simulink model "HVModAL_Fahrzeugmodell"  (R2015b)
settings: Solver=ode1  StartTime=0  StopTime=drp.driving_cycle.tstop  FixedStep=sim_params.Ts  RelTol=1e-5
PreLoadFcn:
  | % Add paths
  | addpath data
  | addpath(genpath('library'))
StartFcn:
  | Simulation.StartTime = tic;
StopFcn:
  | Simulation.DurationTime = toc(Simulation.StartTime);
undefined symbols (not defined in the file or in its folder): Batteries, BMS, BMS_Bat_, C_Nenn_DCDC1, C_Nenn_DCDC2, d2d, DC, DCDC_Converter_efficiency, DcDc_Converters, Dcl, drp, drv, elm, gen, gin, Hdc, hdc, HV, hvb, Hvb, ice, ldc, lib_dcl, lib_hdc, lib_hvb, lib_veh, Link, lossestable, mask_LUT_OCV, mask_LUT_OCV_SOC, mask_LUT_OCV_Temperature, mask_LUT_R, mask_LUT_Rs, mask_LUT_Rs_SOC, mask_LUT_Rs_Temperature, sim_params, speedvec, torquevec, tri, veh, Veh, Vehicle_Chassis
libraries: simulink x29, lib_tri_modules x7, lib_hdc_module x5, lib_gearbox x4, lib_hvb_battery_pack x3, cstblocks x3, PowerLimitBlock x2, MultiCellLibrary x2, lib_aux x1, lib_drv x1, lib_gen x1, lib_elm x1
(part 3 of 7)

== system HVModAL_Fahrzeugmodell/Visualization (Vis)/Subsystem1 ==
  Aux Scope : Scope  NumInputPorts=2
  Auxillaries (aux) : Subsystem
  DC-Link (Dcl) : Subsystem
  DC/DC Converter (hdc) : Subsystem
  DC/DC Scope1 : Scope  NumInputPorts=3
  DC/DC Scope2 : Scope  NumInputPorts=4
  Dcl Scope : Scope  NumInputPorts=4
  Degradation1 : Scope  Commented=on  NumInputPorts=8
  Degradation2 : Scope  Commented=on  NumInputPorts=8
  Demux{1..2,4..5} (4 alike) : Demux  Commented=on  Outputs=3
  Demux3 : Demux  Commented=on  Outputs=8
  Driver (Drv) : Subsystem
  Driver Scope : Scope  NumInputPorts=4
  EMS : Subsystem
  Elm : Subsystem
  Elm Scope : Scope  NumInputPorts=3
  Elm Scope1 : Scope  NumInputPorts=3
  Energy-Disppation Bat1+Bat2 : Scope  NumInputPorts=4
  HV-Batteries (hvb) : Subsystem
  HV-Batteries Scope : Scope  NumInputPorts=6
  Hvb Scope : Scope
  Hvb Scope1 : Scope
  LV-DCDC (ldc) : Subsystem
  Ldc Scope 1 : Scope  NumInputPorts=3
  Ldc Scope 2 : Scope  NumInputPorts=3
  Subsystem1 : Subsystem  Commented=on
  Sum of Elements : Sum  Commented=on  Inputs=+
  Sum of Elements1 : Sum  Commented=on  Inputs=+
  Sum of Elements2 : Sum  Commented=on  Inputs=+
  Terminator{,1..7} (8 alike) : Terminator  Commented=on
  Traction Inverters(Tri) : Subsystem
  Traction Inverters(Tri)- Scope : Scope  NumInputPorts=5
  Veh Scope : Scope  NumInputPorts=5
  Veh Scope 2 : Scope  NumInputPorts=4
  Vehicle (veh) : Subsystem
  wires:
  Vehicle (veh)/4(Veh_F_roll) -> Veh Scope/4  "Veh_F_roll"
  LV-DCDC (ldc)/2(Ldc_P_HvBat_vec) -> Ldc Scope 2/2  "Ldc_P_HvBat_vec"
  Elm/1(Elm_T_el_vec) -> Elm Scope/1  "Elm_T_el"
  Elm/3(Elm_P_losses_vec) -> Elm Scope/3  "Elm_P_losses"
  HV-Batteries (hvb)/12(Hvb_Bat1_Plosses) -> Hvb Scope/1
  DC/DC Converter (hdc)/3(Hdc_P_losses_vec) -> DC/DC Scope2/3  "Hdc_P_losses"
  DC/DC Converter (hdc)/5(Hdc_error_vec) -> DC/DC Scope1/1  "Hdc_error"
  DC/DC Converter (hdc)/6(Hdc_Pmax_vec) -> DC/DC Scope1/2  "Hdc_Pmax"
  Elm/2(Elm_P_actual_vec) -> Elm Scope/2  "Elm_P_actual"
  Traction Inverters(Tri)/5(Tri_atJunction) -> Traction Inverters(Tri)- Scope/5  "Tri_atEndwinding"
  Traction Inverters(Tri)/2(Tri_P_losses) -> Traction Inverters(Tri)- Scope/2  "Tri_P_losses"
  DC/DC Converter (hdc)/4(Hdc_fac_eta_vec) -> DC/DC Scope2/4  "Hdc_fac_eta"
  DC/DC Converter (hdc)/2(Hdc_P_dclink_vec) -> DC/DC Scope2/2  "Hdc_P_dclink"
  HV-Batteries (hvb)/7(Hvb_Bat2_P) -> HV-Batteries Scope/5  "Hvb_Bat2_P"
  HV-Batteries (hvb)/8(Hvb_Bat2_SOC) -> HV-Batteries Scope/6  "Hvb_Bat2_SOC"
  Vehicle (veh)/2(Veh_F_climb) -> Veh Scope/2  "Veh_F_climb"
  Auxillaries (aux)/1(Aux_P_lv_bat) -> Aux Scope/1  "Aux_P_lv_bat"
  HV-Batteries (hvb)/5(Hvb_Bat2_U) -> HV-Batteries Scope/4  "Hvb_Bat2_U"
  HV-Batteries (hvb)/3(Hvb_Bat1_P) -> HV-Batteries Scope/2  "Hvb_Bat1_P"
  HV-Batteries (hvb)/4(Hvb_Bat1_SOC) -> HV-Batteries Scope/3  "Hvb_Bat1_SOC"
  Traction Inverters(Tri)/4(Tri_Pmax) -> Traction Inverters(Tri)- Scope/4  "Tri_Pmax"
  DC-Link (Dcl)/3(Dcl_P_totalwoHdcPdc) -> Dcl Scope/3  "Dcl_P_totalwoHdcPdc"
  HV-Batteries (hvb)/1(Hvb_Bat1_U) -> HV-Batteries Scope/1  "Hvb_Bat1_U"
  Auxillaries (aux)/2(Aux_P_dcLink) -> Aux Scope/2  "Aux_P_dcLink"
  Driver (Drv)/1(fac_pedAcc) -> Driver Scope/1  "fac_pedAcc"
  Vehicle (veh)/3(Veh_F_drive) -> Veh Scope/3  "Veh_F_drive"
  Traction Inverters(Tri)/3(Tri_eta) -> Traction Inverters(Tri)- Scope/3  "Tri_eta"
  LV-DCDC (ldc)/5(Ldc_Pmax_vec) -> Ldc Scope 1/2  "Ldc_Pmax_vec"
  DC/DC Converter (hdc)/1(Hdc_P_bat_vec) -> DC/DC Scope2/1  "Hdc_P_bat"
  LV-DCDC (ldc)/4(Ldc_atJunction_vec) -> Ldc Scope 1/1  "Ldc_atJunction_vec"
  Vehicle (veh)/1(Veh_F_aero) -> Veh Scope/1  "Veh_F_aero"
  Vehicle (veh)/5(Veh_F_acc) -> Veh Scope 2/1, Veh Scope/5  "Veh_F_acc"
  Vehicle (veh)/7(Veh_v_actual) -> Veh Scope 2/3
  Elm/4(Elm1_I_abc) -> Elm Scope1/1  "Elm1_I_abc"
  Elm/6(Elm_at_endWindingsMagnet_vec) -> Elm Scope1/3  "at_end_windingsMagnet_vec"
  Vehicle (veh)/6(Veh_a_actual) -> Veh Scope 2/2
  Vehicle (veh)/8(Veh_v_actual-v_wheel) -> Veh Scope 2/4
  DC-Link (Dcl)/4(Hdc_P_dcLink) -> Dcl Scope/4  "Hdc_P_dcLink"
  DC-Link (Dcl)/1(Dcl_U) -> Dcl Scope/1  "Dcl_U"
  LV-DCDC (ldc)/3(Ldc_P_dcLink) -> Ldc Scope 2/3  "Ldc_P_dcLink"
  LV-DCDC (ldc)/6(Ldc_error_vec) -> Ldc Scope 1/3  "Ldc_error_vec"
  Traction Inverters(Tri)/1(Tri_P_dcLink) -> Traction Inverters(Tri)- Scope/1  "Tri_P_dcLink"
  LV-DCDC (ldc)/1(Ldc_P_Lv_bat) -> Ldc Scope 2/1  "LdcP_Lv_bat"
  Elm/5(Elm_Pmax_vec) -> Elm Scope1/2  "Elm_Pmax_vec"
  DC/DC Converter (hdc)/7(Hdc_at_Junction_vec) -> DC/DC Scope1/3
  Driver (Drv)/2(Emg_T_el_demand) -> Driver Scope/2  "Emg_T_el_demand"
  Driver (Drv)/3(Emg_T_mech_demand) -> Driver Scope/3  "Emg_T_mech_demand"
  DC-Link (Dcl)/2(Dcl_P_total) -> Dcl Scope/2  "Dcl_P_total"
  Driver (Drv)/4(v_cycle(km/h)) -> Driver Scope/4
  EMS/1(Emg_fac_powerDristri_Bat1) -> Energy-Disppation Bat1+Bat2/1  "Emg_fac_powerDristri_Bat1"
  EMS/2(Emg_fac_powerDristri_Bat2) -> Energy-Disppation Bat1+Bat2/2  "Emg_fac_powerDristri_Bat2"
  EMS/6(Emg_T_elDemand_Inv1) -> Energy-Disppation Bat1+Bat2/3  "Emg_T_elDemand_Inv1"
  EMS/7(Emg_T_elDemand_Inv2) -> Energy-Disppation Bat1+Bat2/4  "Emg_T_elDemand_Inv2"
  Vehicle (veh)/9(Veh_Ploss_gearbox) -> Hvb Scope1/1  "Veh_Ploss_gearbox"
  Demux3/1 -> Terminator5/1  "elm1_mot"
  EMS/8(Emg_Degradation) -> Demux3/1
  Demux3/2 -> Terminator4/1  "elm1_gen"
  Demux1/1 -> Sum of Elements/1
  Demux1/2 -> Sum of Elements1/1
  Demux1/3 -> Sum of Elements2/1
  Demux4/1 -> Degradation1/5
  Demux4/2 -> Degradation1/6
  Demux4/3 -> Degradation1/7
  Subsystem1/1(v_deviation(km/h)) -> Degradation2/4, Degradation2/8, Degradation1/4, Degradation1/8
  Demux3/3 -> Terminator6/1  "elm1_mot"
  Demux3/4 -> Terminator7/1  "elm1_gen"
  Demux2/1 -> Degradation2/1
  Demux2/2 -> Degradation2/2
  Demux2/3 -> Degradation2/3
  Demux5/1 -> Degradation2/5
  Demux5/2 -> Degradation2/6
  Demux5/3 -> Degradation2/7
  Sum of Elements/1 -> Degradation1/1
  Sum of Elements1/1 -> Degradation1/2
  Sum of Elements2/1 -> Degradation1/3
  Demux3/5 -> Terminator/1  "tri1_gen"
  Demux3/6 -> Terminator1/1  "DC-Link_gen"
  Demux3/7 -> Terminator2/1
  Demux3/8 -> Terminator3/1

== system HVModAL_Fahrzeugmodell/Energy Manager (Emg)/Battery Control/Driving_Mode ==
  SB_BMS_1 : Inport
  SB_BMS_2 : Inport  Port=2
  SB_BMS_3 : Inport  Port=3
  Veh_v_actual : Inport  Port=4
  Tri_BusSW : Inport  Port=5
  "Aux_BusSW " : Inport  Port=6
  Enable : EnablePort
  Merge : Merge  Inputs=5
  Range_extender 1 : Subsystem  Commented=on  TreatAsAtomicUnit=on
  Range_extender 2 : Subsystem  TreatAsAtomicUnit=on
  Strategy_Maximiziation_Available_Batterypower : Subsystem  TreatAsAtomicUnit=on
  Strategy_Maximiziation_Driving_Range1 : Subsystem  Commented=on  TreatAsAtomicUnit=on
  Strategy_Minimization_Current_Trip_Costs : Subsystem  TreatAsAtomicUnit=on
  Strategy_Minimization_LifeCycleCosts : Subsystem  TreatAsAtomicUnit=on
  Switch Case : SwitchCase  CaseConditions={2, 3, 4,5}
  n_Power_Distribution_Strategy : Constant  Value=5
  vector_PowerDistribution : Outport
  case : Outport  Port=2
  I_rex : Outport  Port=3
  wires:
  Merge/1 -> vector_PowerDistribution/1
  Switch Case/1 -> Strategy_Minimization_Current_Trip_Costs/Action
  Switch Case/2 -> Strategy_Minimization_LifeCycleCosts/Action
  Switch Case/3 -> Strategy_Maximiziation_Driving_Range1/Action
  Switch Case/5 -> Strategy_Maximiziation_Available_Batterypower/Action
  SB_BMS_3/1 -> Range_extender 2/3(SB_BMS_3), Strategy_Maximiziation_Driving_Range1/3(SB_BMS_3), Strategy_Maximiziation_Available_Batterypower/3(SB_BMS_3)
  SB_BMS_2/1 -> Range_extender 2/2(SB_BMS_2), Strategy_Maximiziation_Driving_Range1/2(SB_BMS_2), Strategy_Maximiziation_Available_Batterypower/2(SB_BMS_2)
  SB_BMS_1/1 -> Range_extender 2/1(SB_BMS_1), Strategy_Maximiziation_Driving_Range1/1(SB_BMS_1), Strategy_Maximiziation_Available_Batterypower/1(SB_BMS_1)
  n_Power_Distribution_Strategy/1 -> case/1, Switch Case/1
  Strategy_Minimization_LifeCycleCosts/1(vector_PowerDistribution) -> Merge/3
  Strategy_Maximiziation_Available_Batterypower/1(vector_PowerDistribution) -> Merge/1
  Strategy_Maximiziation_Driving_Range1/1(vector_PowerDistribution) -> Merge/4
  Strategy_Minimization_Current_Trip_Costs/1(vector_PowerDistribution) -> Merge/2
  ? -> ?
  Switch Case/4 -> Range_extender 2/Action
  Range_extender 2/1(vector_PowerDistribution) -> Merge/5
  Veh_v_actual/1 -> Range_extender 2/4(Veh_v_actual)
  Range_extender 2/2(I_rex) -> I_rex/1
  Tri_BusSW/1 -> Range_extender 2/5(Tri_BusSW)
  "Aux_BusSW "/1 -> Range_extender 2/6("Aux_BusSW ")

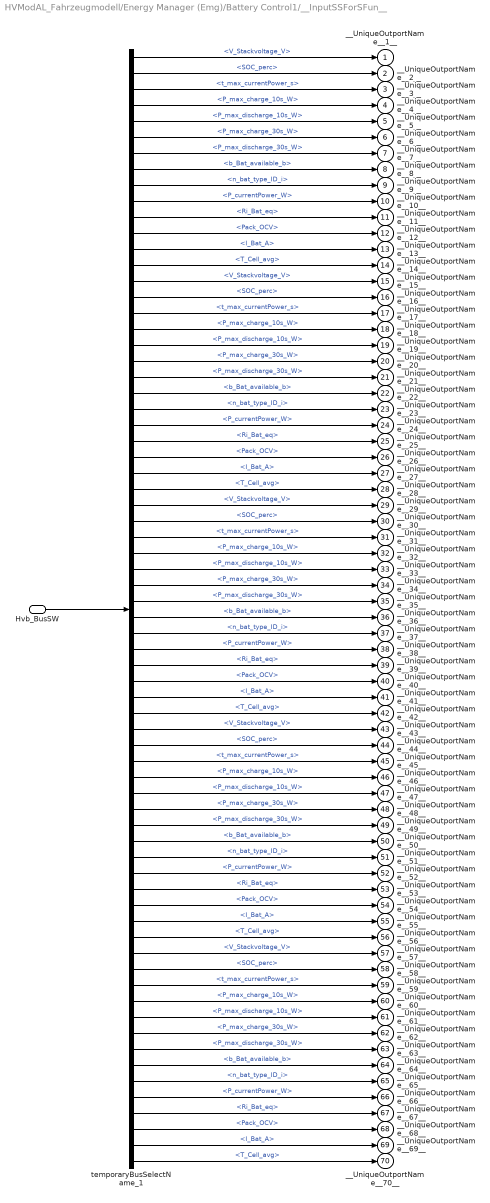
== system HVModAL_Fahrzeugmodell/Energy Manager (Emg)/Battery Control1/__InputSSForSFun__ ==
  Hvb_BusSW : Inport
  temporaryBusSelectName_1 : BusSelector  OutputSignals=SB_Bat1.V_Stackvoltage_V,SB_Bat1.SOC_perc,SB_Bat1.t_max_currentPower_s,SB_Bat1.P_max_charge_10s_W,SB_Bat1.P_max_discharge_10s_W,SB_Bat1.P_max_charge_30s_W,SB_Bat1.P_max_discharge_30s_W,SB_Bat1.b_Bat_available_b,SB_Bat1.n_bat_type_ID_i,SB_Bat1.P_currentPower_W,SB_Bat1.Ri_Bat_eq,SB_Bat1.Pack_OCV,SB_Bat1.I_Bat_A,SB_Bat1.T_Cell_avg,SB_Bat2.V_Stackvoltage_V,SB_Bat2.SOC_perc,SB_Bat2.t_max_currentPower_s,SB_Bat2.P_max_charge_10s_W,SB_Bat2.P_max_discharge_10s_W,SB_Bat2.P_max_charge_30s_W,SB_Bat2.P_max_discharge_30s_W,SB_Bat2.b_Bat_available_b,SB_Bat2.n_bat_type_ID_i,SB_Bat2.P_currentPower_W,SB_Bat2.Ri_Bat_eq,SB_Bat2.Pack_OCV,SB_Bat2.I_Bat_A,SB_Bat2.T_Cell_avg,SB_Bat3.V_Stackvoltage_V,SB_Bat3.SOC_perc,SB_Bat3.t_max_currentPower_s,SB_Bat3.P_max_charge_10s_W,SB_Bat3.P_max_discharge_10s_W,SB_Bat3.P_max_charge_30s_W,SB_Bat3.P_max_discharge_30s_W,SB_Bat3.b_Bat_available_b,SB_Bat3.n_bat_type_ID_i,SB_Bat3.P_currentPower_W,SB_Bat3.Ri_Bat_eq,SB_Bat3.Pack_OCV,SB_Bat3.I_Bat_A,SB_Bat3.T_Cell_avg,SB_Bat4.V_Stackvoltage_V,SB_Bat4.SOC_perc,SB_Bat4.t_max_currentPower_s,SB_Bat4.P_max_charge_10s_W,SB_Bat4.P_max_discharge_10s_W,SB_Bat4.P_max_charge_30s_W,SB_Bat4.P_max_discharge_30s_W,SB_Bat4.b_Bat_available_b,SB_Bat4.n_bat_type_ID_i,SB_Bat4.P_currentPower_W,SB_Bat4.Ri_Bat_eq,SB_Bat4.Pack_OCV,SB_Bat4.I_Bat_A,SB_Bat4.T_Cell_avg,SB_Bat5.V_Stackvoltage_V,SB_Bat5.SOC_perc,SB_Bat5.t_max_currentPower_s,SB_Bat5.P_max_charge_10s_W,SB_Bat5.P_max_discharge_10s_W,SB_Bat5.P_max_charge_30s_W,SB_Bat5.P_max_discharge_30s_W,SB_Bat5.b_Bat_available_b,SB_Bat5.n_bat_type_ID_i,SB_Bat5.P_currentPower_W,SB_Bat5.Ri_Bat_eq,SB_Bat5.Pack_OCV,SB_Bat5.I_Bat_A,SB_Bat5.T_Cell_avg
  __UniqueOutportName__1__ : Outport
  __UniqueOutportName__2__ : Outport  Port=2
  __UniqueOutportName__3__ : Outport  Port=3
  __UniqueOutportName__4__ : Outport  Port=4
  __UniqueOutportName__5__ : Outport  Port=5
  __UniqueOutportName__6__ : Outport  Port=6
  __UniqueOutportName__7__ : Outport  Port=7
  __UniqueOutportName__8__ : Outport  Port=8
  __UniqueOutportName__9__ : Outport  Port=9
  __UniqueOutportName__10__ : Outport  Port=10
  __UniqueOutportName__11__ : Outport  Port=11
  __UniqueOutportName__12__ : Outport  Port=12
  __UniqueOutportName__13__ : Outport  Port=13
  __UniqueOutportName__14__ : Outport  Port=14
  __UniqueOutportName__15__ : Outport  Port=15
  __UniqueOutportName__16__ : Outport  Port=16
  __UniqueOutportName__17__ : Outport  Port=17
  __UniqueOutportName__18__ : Outport  Port=18
  __UniqueOutportName__19__ : Outport  Port=19
  __UniqueOutportName__20__ : Outport  Port=20
  __UniqueOutportName__21__ : Outport  Port=21
  __UniqueOutportName__22__ : Outport  Port=22
  __UniqueOutportName__23__ : Outport  Port=23
  __UniqueOutportName__24__ : Outport  Port=24
  __UniqueOutportName__25__ : Outport  Port=25
  __UniqueOutportName__26__ : Outport  Port=26
  __UniqueOutportName__27__ : Outport  Port=27
  __UniqueOutportName__28__ : Outport  Port=28
  __UniqueOutportName__29__ : Outport  Port=29
  __UniqueOutportName__30__ : Outport  Port=30
  __UniqueOutportName__31__ : Outport  Port=31
  __UniqueOutportName__32__ : Outport  Port=32
  __UniqueOutportName__33__ : Outport  Port=33
  __UniqueOutportName__34__ : Outport  Port=34
  __UniqueOutportName__35__ : Outport  Port=35
  __UniqueOutportName__36__ : Outport  Port=36
  __UniqueOutportName__37__ : Outport  Port=37
  __UniqueOutportName__38__ : Outport  Port=38
  __UniqueOutportName__39__ : Outport  Port=39
  __UniqueOutportName__40__ : Outport  Port=40
  __UniqueOutportName__41__ : Outport  Port=41
  __UniqueOutportName__42__ : Outport  Port=42
  __UniqueOutportName__43__ : Outport  Port=43
  __UniqueOutportName__44__ : Outport  Port=44
  __UniqueOutportName__45__ : Outport  Port=45
  __UniqueOutportName__46__ : Outport  Port=46
  __UniqueOutportName__47__ : Outport  Port=47
  __UniqueOutportName__48__ : Outport  Port=48
  __UniqueOutportName__49__ : Outport  Port=49
  __UniqueOutportName__50__ : Outport  Port=50
  __UniqueOutportName__51__ : Outport  Port=51
  __UniqueOutportName__52__ : Outport  Port=52
  __UniqueOutportName__53__ : Outport  Port=53
  __UniqueOutportName__54__ : Outport  Port=54
  __UniqueOutportName__55__ : Outport  Port=55
  __UniqueOutportName__56__ : Outport  Port=56
  __UniqueOutportName__57__ : Outport  Port=57
  __UniqueOutportName__58__ : Outport  Port=58
  __UniqueOutportName__59__ : Outport  Port=59
  __UniqueOutportName__60__ : Outport  Port=60
  __UniqueOutportName__61__ : Outport  Port=61
  __UniqueOutportName__62__ : Outport  Port=62
  __UniqueOutportName__63__ : Outport  Port=63
  __UniqueOutportName__64__ : Outport  Port=64
  __UniqueOutportName__65__ : Outport  Port=65
  __UniqueOutportName__66__ : Outport  Port=66
  __UniqueOutportName__67__ : Outport  Port=67
  __UniqueOutportName__68__ : Outport  Port=68
  __UniqueOutportName__69__ : Outport  Port=69
  __UniqueOutportName__70__ : Outport  Port=70
  wires:
  Hvb_BusSW/1 -> temporaryBusSelectName_1/1
  temporaryBusSelectName_1/1 -> __UniqueOutportName__1__/1  "<V_Stackvoltage_V>"
  temporaryBusSelectName_1/2 -> __UniqueOutportName__2__/1  "<SOC_perc>"
  temporaryBusSelectName_1/3 -> __UniqueOutportName__3__/1  "<t_max_currentPower_s>"
  temporaryBusSelectName_1/4 -> __UniqueOutportName__4__/1  "<P_max_charge_10s_W>"
  temporaryBusSelectName_1/5 -> __UniqueOutportName__5__/1  "<P_max_discharge_10s_W>"
  temporaryBusSelectName_1/6 -> __UniqueOutportName__6__/1  "<P_max_charge_30s_W>"
  temporaryBusSelectName_1/7 -> __UniqueOutportName__7__/1  "<P_max_discharge_30s_W>"
  temporaryBusSelectName_1/8 -> __UniqueOutportName__8__/1  "<b_Bat_available_b>"
  temporaryBusSelectName_1/9 -> __UniqueOutportName__9__/1  "<n_bat_type_ID_i>"
  temporaryBusSelectName_1/10 -> __UniqueOutportName__10__/1  "<P_currentPower_W>"
  temporaryBusSelectName_1/11 -> __UniqueOutportName__11__/1  "<Ri_Bat_eq>"
  temporaryBusSelectName_1/12 -> __UniqueOutportName__12__/1  "<Pack_OCV>"
  temporaryBusSelectName_1/13 -> __UniqueOutportName__13__/1  "<I_Bat_A>"
  temporaryBusSelectName_1/14 -> __UniqueOutportName__14__/1  "<T_Cell_avg>"
  temporaryBusSelectName_1/15 -> __UniqueOutportName__15__/1  "<V_Stackvoltage_V>"
  temporaryBusSelectName_1/16 -> __UniqueOutportName__16__/1  "<SOC_perc>"
  temporaryBusSelectName_1/17 -> __UniqueOutportName__17__/1  "<t_max_currentPower_s>"
  temporaryBusSelectName_1/18 -> __UniqueOutportName__18__/1  "<P_max_charge_10s_W>"
  temporaryBusSelectName_1/19 -> __UniqueOutportName__19__/1  "<P_max_discharge_10s_W>"
  temporaryBusSelectName_1/20 -> __UniqueOutportName__20__/1  "<P_max_charge_30s_W>"
  temporaryBusSelectName_1/21 -> __UniqueOutportName__21__/1  "<P_max_discharge_30s_W>"
  temporaryBusSelectName_1/22 -> __UniqueOutportName__22__/1  "<b_Bat_available_b>"
  temporaryBusSelectName_1/23 -> __UniqueOutportName__23__/1  "<n_bat_type_ID_i>"
  temporaryBusSelectName_1/24 -> __UniqueOutportName__24__/1  "<P_currentPower_W>"
  temporaryBusSelectName_1/25 -> __UniqueOutportName__25__/1  "<Ri_Bat_eq>"
  temporaryBusSelectName_1/26 -> __UniqueOutportName__26__/1  "<Pack_OCV>"
  temporaryBusSelectName_1/27 -> __UniqueOutportName__27__/1  "<I_Bat_A>"
  temporaryBusSelectName_1/28 -> __UniqueOutportName__28__/1  "<T_Cell_avg>"
  temporaryBusSelectName_1/29 -> __UniqueOutportName__29__/1  "<V_Stackvoltage_V>"
  temporaryBusSelectName_1/30 -> __UniqueOutportName__30__/1  "<SOC_perc>"
  temporaryBusSelectName_1/31 -> __UniqueOutportName__31__/1  "<t_max_currentPower_s>"
  temporaryBusSelectName_1/32 -> __UniqueOutportName__32__/1  "<P_max_charge_10s_W>"
  temporaryBusSelectName_1/33 -> __UniqueOutportName__33__/1  "<P_max_discharge_10s_W>"
  temporaryBusSelectName_1/34 -> __UniqueOutportName__34__/1  "<P_max_charge_30s_W>"
  temporaryBusSelectName_1/35 -> __UniqueOutportName__35__/1  "<P_max_discharge_30s_W>"
  temporaryBusSelectName_1/36 -> __UniqueOutportName__36__/1  "<b_Bat_available_b>"
  temporaryBusSelectName_1/37 -> __UniqueOutportName__37__/1  "<n_bat_type_ID_i>"
  temporaryBusSelectName_1/38 -> __UniqueOutportName__38__/1  "<P_currentPower_W>"
  temporaryBusSelectName_1/39 -> __UniqueOutportName__39__/1  "<Ri_Bat_eq>"
  temporaryBusSelectName_1/40 -> __UniqueOutportName__40__/1  "<Pack_OCV>"
  temporaryBusSelectName_1/41 -> __UniqueOutportName__41__/1  "<I_Bat_A>"
  temporaryBusSelectName_1/42 -> __UniqueOutportName__42__/1  "<T_Cell_avg>"
  temporaryBusSelectName_1/43 -> __UniqueOutportName__43__/1  "<V_Stackvoltage_V>"
  temporaryBusSelectName_1/44 -> __UniqueOutportName__44__/1  "<SOC_perc>"
  temporaryBusSelectName_1/45 -> __UniqueOutportName__45__/1  "<t_max_currentPower_s>"
  temporaryBusSelectName_1/46 -> __UniqueOutportName__46__/1  "<P_max_charge_10s_W>"
  temporaryBusSelectName_1/47 -> __UniqueOutportName__47__/1  "<P_max_discharge_10s_W>"
  temporaryBusSelectName_1/48 -> __UniqueOutportName__48__/1  "<P_max_charge_30s_W>"
  temporaryBusSelectName_1/49 -> __UniqueOutportName__49__/1  "<P_max_discharge_30s_W>"
  temporaryBusSelectName_1/50 -> __UniqueOutportName__50__/1  "<b_Bat_available_b>"
  temporaryBusSelectName_1/51 -> __UniqueOutportName__51__/1  "<n_bat_type_ID_i>"
  temporaryBusSelectName_1/52 -> __UniqueOutportName__52__/1  "<P_currentPower_W>"
  temporaryBusSelectName_1/53 -> __UniqueOutportName__53__/1  "<Ri_Bat_eq>"
  temporaryBusSelectName_1/54 -> __UniqueOutportName__54__/1  "<Pack_OCV>"
  temporaryBusSelectName_1/55 -> __UniqueOutportName__55__/1  "<I_Bat_A>"
  temporaryBusSelectName_1/56 -> __UniqueOutportName__56__/1  "<T_Cell_avg>"
  temporaryBusSelectName_1/57 -> __UniqueOutportName__57__/1  "<V_Stackvoltage_V>"
  temporaryBusSelectName_1/58 -> __UniqueOutportName__58__/1  "<SOC_perc>"
  temporaryBusSelectName_1/59 -> __UniqueOutportName__59__/1  "<t_max_currentPower_s>"
  temporaryBusSelectName_1/60 -> __UniqueOutportName__60__/1  "<P_max_charge_10s_W>"
  temporaryBusSelectName_1/61 -> __UniqueOutportName__61__/1  "<P_max_discharge_10s_W>"
  temporaryBusSelectName_1/62 -> __UniqueOutportName__62__/1  "<P_max_charge_30s_W>"
  temporaryBusSelectName_1/63 -> __UniqueOutportName__63__/1  "<P_max_discharge_30s_W>"
  temporaryBusSelectName_1/64 -> __UniqueOutportName__64__/1  "<b_Bat_available_b>"
  temporaryBusSelectName_1/65 -> __UniqueOutportName__65__/1  "<n_bat_type_ID_i>"
  temporaryBusSelectName_1/66 -> __UniqueOutportName__66__/1  "<P_currentPower_W>"
  temporaryBusSelectName_1/67 -> __UniqueOutportName__67__/1  "<Ri_Bat_eq>"
  temporaryBusSelectName_1/68 -> __UniqueOutportName__68__/1  "<Pack_OCV>"
  temporaryBusSelectName_1/69 -> __UniqueOutportName__69__/1  "<I_Bat_A>"
  temporaryBusSelectName_1/70 -> __UniqueOutportName__70__/1  "<T_Cell_avg>"

== system HVModAL_Fahrzeugmodell/Energy Manager (Emg)/Battery Control1/__OutputSSForSFun__ ==
  __UniqueInportName__1__ : Inport
  Emg_fac_powerDistribution_vec : Outport
  wires:
  __UniqueInportName__1__/1 -> Emg_fac_powerDistribution_vec/1  "Emg_fac_powerDistribution_vec"

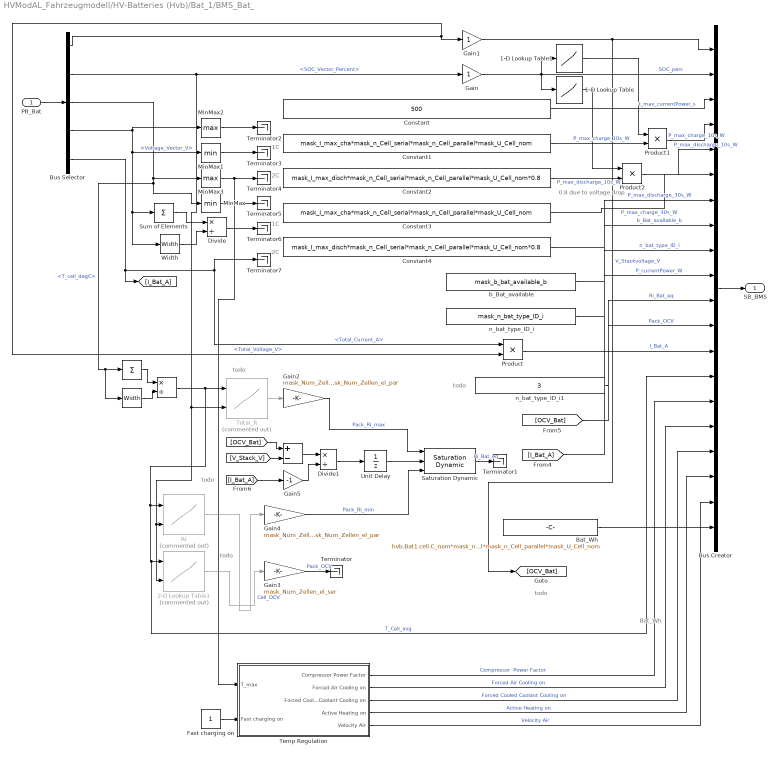
== system HVModAL_Fahrzeugmodell/HV-Batteries (Hvb)/Bat_1/BMS_Bat_ ==
  note: Bat_Wh
  note: 0.8 due to voltage drop
  note: todo
  note: 1C
  note: 2C
  note: 1C
  note: 2C
  note: todo
  note: todo
  note: todo
  note: todo
  PB_Bat : Inport
  " " : Product  Inputs=*/
  " " : Sum  Inputs=+
  " " : Width
  " " : Sum  Inputs=+-
  1-D Lookup Table : Lookup_n-D  NumberOfTableDimensions=1  BreakpointsForDimension1=[0,10,20,40,60,80,100]  Table=[0,0.5,0.8,1,1,1,1]  InternalRulePriority=Speed  RndMeth=Simplest  InputSameDT=on
  1-D Lookup Table1 : Lookup_n-D  NumberOfTableDimensions=1  BreakpointsForDimension1=[0 20 40 60 80 100]  Table=[1 1 1 1 0.7 0]  InternalRulePriority=Speed  RndMeth=Simplest  InputSameDT=on
  2-D Lookup Table1 : Lookup_n-D  Commented=on  BreakpointsForDimension1=mask_LUT_OCV_Temperature  BreakpointsForDimension2=mask_LUT_OCV_SOC  Table=mask_LUT_OCV  InternalRulePriority=Speed  RndMeth=Simplest  InputSameDT=on
  Bat_Wh : Constant  Value=hvb.Bat1.cell.C_nom*mask_n_Cell_serial*mask_n_Cell_parallel*mask_U_Cell_nom
  Bus Creator : BusCreator  Inputs=20
  Bus Selector : BusSelector  OutputSignals=Total_Voltage_V,SOC_Vector_Percent,T_cell_degC,Voltage_Vector_V,Total_Current_A
  Constant : Constant  Value=500
  Constant1 : Constant  Value=mask_I_max_cha*mask_n_Cell_serial*mask_n_Cell_parallel*mask_U_Cell_nom
  Constant2 : Constant  Value=mask_I_max_disch*mask_n_Cell_serial*mask_n_Cell_parallel*mask_U_Cell_nom*0.8
  Constant3 : Constant  Value=mask_I_max_cha*mask_n_Cell_serial*mask_n_Cell_parallel*mask_U_Cell_nom
  Constant4 : Constant  Value=mask_I_max_disch*mask_n_Cell_serial*mask_n_Cell_parallel*mask_U_Cell_nom*0.8
  Divide : Product  Inputs=*/
  Divide1 : Product  Inputs=*/
  Fast charging on : Constant
  Gain : Gain
  Gain1 : Gain
  Gain2 : Gain  Gain=mask_Num_Zellen_el_ser/mask_Num_Zellen_el_par
  Gain3 : Gain  Gain=mask_Num_Zellen_el_ser
  Gain4 : Gain  Gain=mask_Num_Zellen_el_ser/mask_Num_Zellen_el_par
  Gain5 : Gain  Gain=-1
  MinMax : MinMax
  MinMax1 : MinMax
  MinMax2 : MinMax  Function=max
  MinMax3 : MinMax  Function=max
  Product : Product  RndMeth=Zero
  Product1 : Product  RndMeth=Zero
  Product2 : Product  RndMeth=Zero
  Ri : Lookup_n-D  Commented=on  BreakpointsForDimension1=mask_LUT_Rs_Temperature  BreakpointsForDimension2=mask_LUT_Rs_SOC  Table=mask_LUT_Rs  InternalRulePriority=Speed  RndMeth=Simplest  InputSameDT=on
  Saturation Dynamic : simulink/Discontinuities/Saturation Dynamic  OutMin=[]  OutMax=[]  OutDataTypeStr=Inherit: Same as second input  OutDataType=fixdt(1, 16)  OutScaling=2^-10  DoSatur=off
  Sum of Elements : Sum  Inputs=+
  Temp Regulation : Subsystem
  Terminator{,1..7} (8 alike) : Terminator
  Total_R : Lookup_n-D  Commented=on  BreakpointsForDimension1=mask_LUT_Rs_Temperature  BreakpointsForDimension2=mask_LUT_Rs_SOC  Table=mask_LUT_R  InternalRulePriority=Speed  RndMeth=Simplest  InputSameDT=on
  Unit Delay : UnitDelay  InitialCondition=0.1  SampleTime=-1
  Width : Width
  b_Bat_available : Constant  Value=mask_b_bat_available_b
  n_bat_type_ID_i : Constant  Value=mask_n_bat_type_ID_i
  n_bat_type_ID_i1 : Constant  Value=3
  SB_BMS : Outport
  wires:
  Gain1/1 -> [OCV_Bat], Bus Creator/1  "V_Stackvoltage_V"
  n_bat_type_ID_i/1 -> Bus Creator/9  "n_bat_type_ID_i"
  b_Bat_available/1 -> Bus Creator/8  "b_Bat_available_b"
  Constant4/1 -> Bus Creator/7  "P_max_discharge_30s_W"
  Constant3/1 -> Bus Creator/6  "P_max_charge_30s_W"
  Constant2/1 -> Product2/2  "P_max_discharge_10s_W"
  Constant1/1 -> Product1/2  "P_max_charge_10s_W"
  Constant/1 -> Bus Creator/3  "t_max_currentPower_s"
  Bus Selector/5 -> [I_Bat_A], Terminator7/1, Product/1  "<Total_Current_A>"
  Bus Selector/4 -> MinMax2/1, MinMax1/1, Sum of Elements/1, Width/1  "<Voltage_Vector_V>"
  Bus Selector/3 -> " "/1, " "/1, MinMax/1, MinMax3/1  "<T_cell_degC>"
  Bus Selector/1 -> Gain1/1, Product/2  "<Total_Voltage_V>"
  Divide/1 -> Terminator6/1
  Width/1 -> Divide/2
  Sum of Elements/1 -> Divide/1
  MinMax3/1 -> Temp Regulation/1(T_max), Terminator4/1
  MinMax2/1 -> Terminator2/1
  MinMax1/1 -> Terminator3/1
  MinMax/1 -> Terminator5/1
  Gain/1 -> 1-D Lookup Table/1, 1-D Lookup Table1/1, Bus Creator/2  "SOC_perc"
  Bus Creator/1 -> SB_BMS/1
  PB_Bat/1 -> Bus Selector/1
  Product/1 -> Bus Creator/10  "P_currentPower_W"
  Unit Delay/1 -> Saturation Dynamic/2
  [OCV_Bat] -> Bus Creator/12  "Pack_OCV"
  Saturation Dynamic/1 -> Terminator1/1  "Ri_Bat_eq"
  Gain5/1 -> Divide1/2
  " "/1 -> Divide1/1
  [V_Stack_V] -> " "/2
  [OCV_Bat] -> " "/1
  [I_Bat_A] -> Gain5/1
  Divide1/1 -> Unit Delay/1
  [I_Bat_A] -> Bus Creator/13  "I_Bat_A"
  Gain4/1 -> Saturation Dynamic/3  "Pack_Ri_min"
  Ri/1 -> Gain4/1
  Gain3/1 -> Terminator/1  "Pack_OCV"
  Gain2/1 -> Saturation Dynamic/1  "Pack_Ri_max"
  " "/1 -> Ri/1, Bus Creator/14, 2-D Lookup Table1/1, Total_R/1  "T_Cell_avg"
  2-D Lookup Table1/1 -> Gain3/1  "Cell_OCV"
  Total_R/1 -> Gain2/1
  Bus Selector/2 -> Ri/2, 2-D Lookup Table1/2, Total_R/2, Gain/1  "<SOC_Vector_Percent>"
  " "/1 -> " "/2
  " "/1 -> " "/1
  n_bat_type_ID_i1/1 -> Bus Creator/11  "Ri_Bat_eq"
  Product1/1 -> Bus Creator/4  "P_max_charge_10s_W"
  Product2/1 -> Bus Creator/5  "P_max_discharge_10s_W"
  1-D Lookup Table1/1 -> Product1/1
  1-D Lookup Table/1 -> Product2/1
  Temp Regulation/2(Forced Air Cooling on) -> Bus Creator/16  "Forced Air Cooling on"
  Temp Regulation/3(Forced Cooled Coolant Cooling on) -> Bus Creator/17  "Forced Cooled Coolant Cooling on"
  Fast charging on/1 -> Temp Regulation/2(Fast charging on)
  Temp Regulation/4(Active Heating on) -> Bus Creator/18  "Active Heating on"
  Temp Regulation/1(Compressor Power Factor) -> Bus Creator/15  "Compressor  Power Factor"
  Temp Regulation/5(Velocity Air) -> Bus Creator/19  "Velocity Air"
  Bat_Wh/1 -> Bus Creator/20

== system HVModAL_Fahrzeugmodell/HV-Batteries (Hvb)/Bat_1/Temp_model ==
  note: 0: No cooling
      | 1: Active Aircooling
      | 2: Refrigerant Cooling
      | 3: Liquid Cooling
      | 4:Passive Aircooling
  Q_dotLoss : Inport
  T_environment : Inport  Port=2
  ForcedAir Cooling on : Inport  Port=3
  Forced Cooled Coolant Cooling on : Inport  Port=4
  Active Heating on : Inport  Port=5
  Compressor Power Factor : Inport  Port=6
  Velocity Airstream : Inport  Port=7
  ActiveAirCoolingCompressor : Subsystem
  AmbientAir : Subsystem
  Cell : Subsystem
  Cooling system : Constant  Value=mask_cooling_method
  CoolingChannel : Subsystem
  Delay : Delay  DelayLength=1  InitialCondition=0
  Delay1 : Delay  DelayLength=1  InitialCondition=0
  LiquidCoolingCompressor : Subsystem
  Pack2cell : Gain  Gain=1/mask_Num_Zellen_el_ser/mask_Num_Zellen_el_par
  Q_dot Cells2CoolingSys+AmbAir : MultiPortSwitch  DataPortOrder=Zero-based contiguous  Inputs=5
  Q_dot Cells2AmbAir+ Q_dotCells2Refri : Sum
  Q_dotCells2AmbAir+ Q_dotCells2CoolingSys : Sum
  Q_dotCoolantCompr+ Q_dotPTC : Sum
  Q_dot_All_Compressors : Sum
  T_cell  avg : Outport
  Q_dot_ AllCompressors +PTC : Outport  Port=2
  wires:
  Cell/1(T_cell avg) -> T_cell  avg/1, CoolingChannel/2(T_cell avg [K]), AmbientAir/2(T_cell avg)
  T_environment/1 -> CoolingChannel/1(T_environment), AmbientAir/5(T_environment), Cell/2(T_environment)
  LiquidCoolingCompressor/1(Q_dot LiquidCoolingSystem) -> Q_dotCoolantCompr+ Q_dotPTC/1, CoolingChannel/3(Q_dot LiquidCoolingSystem)
  AmbientAir/1(Q_dotHousingDissipation AmbientAir2Environment) -> Delay/1
  ForcedAir Cooling on/1 -> ActiveAirCoolingCompressor/1(ForcedAir Cooling on)
  ActiveAirCoolingCompressor/1(Velocity Air) -> AmbientAir/3(Velocity Air [m/s])
  LiquidCoolingCompressor/2(Q_dot PTC Heater) -> Q_dotCoolantCompr+ Q_dotPTC/2, CoolingChannel/4(Q_dot PTC Heater)
  Q_dot Cells2CoolingSys+AmbAir/1 -> Pack2cell/1  "Q_dot Cells2CoolingSys+AmbAir"
  Cooling system/1 -> Q_dot Cells2CoolingSys+AmbAir/1
  AmbientAir/2(Q_dotCells2AmbientAir) -> Q_dot Cells2CoolingSys+AmbAir/6, Q_dotCells2AmbAir+ Q_dotCells2CoolingSys/1, Q_dot Cells2AmbAir+ Q_dotCells2Refri/1, Q_dot Cells2CoolingSys+AmbAir/3, Q_dot Cells2CoolingSys+AmbAir/2
  CoolingChannel/1(Q_dot Cells2Refri) -> Q_dot Cells2AmbAir+ Q_dotCells2Refri/2
  CoolingChannel/2(Q_dot Cells2CoolingSystem) -> Q_dotCells2AmbAir+ Q_dotCells2CoolingSys/2
  Q_dotLoss/1 -> Cell/3(Q_dot Loss Cell)
  Pack2cell/1 -> Cell/1(Q_dot Cell2CoolingSystem+AmbientAir)  "Q_dot SingleCell2CoolingSys+AmbAir"
  Delay/1 -> AmbientAir/1(Q_dotHousingDissipation AmbientAir2Environment1)
  Q_dotCells2AmbAir+ Q_dotCells2CoolingSys/1 -> Q_dot Cells2CoolingSys+AmbAir/5
  Q_dot Cells2AmbAir+ Q_dotCells2Refri/1 -> Q_dot Cells2CoolingSys+AmbAir/4
  AmbientAir/3(T_AmbientAir) -> Delay1/1
  Delay1/1 -> AmbientAir/6(T_AmbientAir2)
  Forced Cooled Coolant Cooling on/1 -> ActiveAirCoolingCompressor/2(Forced Cooled Coolant Cooling on), LiquidCoolingCompressor/1(Forced Cooled Coolant Cooling on)
  Active Heating on/1 -> LiquidCoolingCompressor/2(Active Heating on)
  Compressor Power Factor/1 -> ActiveAirCoolingCompressor/3(Compressor Power Factor), LiquidCoolingCompressor/3(Compressor Power Factor)
  Velocity Airstream/1 -> ActiveAirCoolingCompressor/4(Velocity Airstream)
  Q_dotCoolantCompr+ Q_dotPTC/1 -> Q_dot_All_Compressors/2
  Q_dot_All_Compressors/1 -> Q_dot_ AllCompressors +PTC/1
  ActiveAirCoolingCompressor/2(Q_dotActiveAirCooling) -> Q_dot_All_Compressors/1, AmbientAir/4(Q_dotActiveAirCooling)

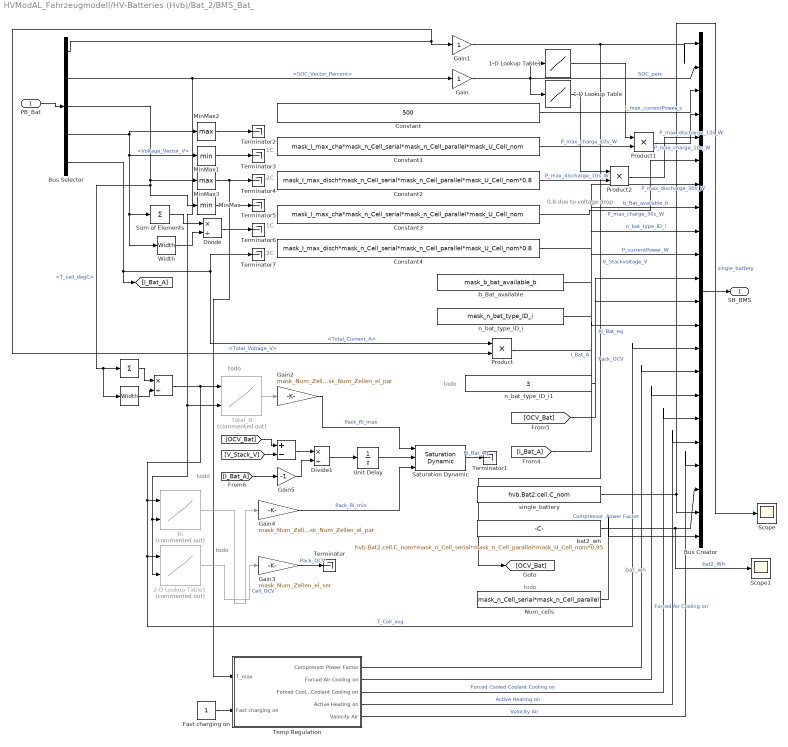
== system HVModAL_Fahrzeugmodell/HV-Batteries (Hvb)/Bat_2/BMS_Bat_ ==
  note: bat_wh
  note: 0.8 due to voltage drop
  note: todo
  note: 1C
  note: 2C
  note: 1C
  note: 2C
  note: todo
  note: todo
  note: todo
  note: todo
  PB_Bat : Inport
  " " : Product  Inputs=*/
  " " : Sum  Inputs=+
  " " : Width
  " " : Sum  Inputs=+-
  1-D Lookup Table : Lookup_n-D  NumberOfTableDimensions=1  BreakpointsForDimension1=[0 10 20 40 60 80 100]  Table=[0 0.2 0.7 0.9 1 1 1]  InternalRulePriority=Speed  RndMeth=Simplest  InputSameDT=on
  1-D Lookup Table1 : Lookup_n-D  NumberOfTableDimensions=1  BreakpointsForDimension1=[0 20 40 60 80 100]  Table=[1 1 1 1 0.7 0]  InternalRulePriority=Speed  RndMeth=Simplest  InputSameDT=on
  2-D Lookup Table1 : Lookup_n-D  Commented=on  BreakpointsForDimension1=mask_LUT_OCV_Temperature  BreakpointsForDimension2=mask_LUT_OCV_SOC  Table=mask_LUT_OCV  InternalRulePriority=Speed  RndMeth=Simplest  InputSameDT=on
  Bus Creator : BusCreator  Inputs=22
  Bus Selector : BusSelector  OutputSignals=Total_Voltage_V,SOC_Vector_Percent,T_cell_degC,Voltage_Vector_V,Total_Current_A
  Constant : Constant  Value=500
  Constant1 : Constant  Value=mask_I_max_cha*mask_n_Cell_serial*mask_n_Cell_parallel*mask_U_Cell_nom
  Constant2 : Constant  Value=mask_I_max_disch*mask_n_Cell_serial*mask_n_Cell_parallel*mask_U_Cell_nom*0.8
  Constant3 : Constant  Value=mask_I_max_cha*mask_n_Cell_serial*mask_n_Cell_parallel*mask_U_Cell_nom
  Constant4 : Constant  Value=mask_I_max_disch*mask_n_Cell_serial*mask_n_Cell_parallel*mask_U_Cell_nom*0.8
  Divide : Product  Inputs=*/
  Divide1 : Product  Inputs=*/
  Fast charging on : Constant
  Gain : Gain
  Gain1 : Gain
  Gain2 : Gain  Gain=mask_Num_Zellen_el_ser/mask_Num_Zellen_el_par
  Gain3 : Gain  Gain=mask_Num_Zellen_el_ser
  Gain4 : Gain  Gain=mask_Num_Zellen_el_ser/mask_Num_Zellen_el_par
  Gain5 : Gain  Gain=-1
  MinMax : MinMax
  MinMax1 : MinMax
  MinMax2 : MinMax  Function=max
  MinMax3 : MinMax  Function=max
  Num_cells : Constant  Value=mask_n_Cell_serial*mask_n_Cell_parallel
  Product : Product  RndMeth=Zero
  Product1 : Product  RndMeth=Zero
  Product2 : Product  RndMeth=Zero
  Ri : Lookup_n-D  Commented=on  BreakpointsForDimension1=mask_LUT_Rs_Temperature  BreakpointsForDimension2=mask_LUT_Rs_SOC  Table=mask_LUT_Rs  InternalRulePriority=Speed  RndMeth=Simplest  InputSameDT=on
  Saturation Dynamic : simulink/Discontinuities/Saturation Dynamic  OutMin=[]  OutMax=[]  OutDataTypeStr=Inherit: Same as second input  OutDataType=fixdt(1, 16)  OutScaling=2^-10  DoSatur=off
  Scope : Scope
  Scope1 : Scope
  Sum of Elements : Sum  Inputs=+
  Temp Regulation : Subsystem
  Terminator{,1..7} (8 alike) : Terminator
  Total_R : Lookup_n-D  Commented=on  BreakpointsForDimension1=mask_LUT_Rs_Temperature  BreakpointsForDimension2=mask_LUT_Rs_SOC  Table=mask_LUT_R  InternalRulePriority=Speed  RndMeth=Simplest  InputSameDT=on
  Unit Delay : UnitDelay  InitialCondition=0.1  SampleTime=-1
  Width : Width
  b_Bat_available : Constant  Value=mask_b_bat_available_b
  bat2_wh : Constant  Value=hvb.Bat2.cell.C_nom*mask_n_Cell_serial*mask_n_Cell_parallel*mask_U_Cell_nom*0.95
  n_bat_type_ID_i : Constant  Value=mask_n_bat_type_ID_i
  n_bat_type_ID_i1 : Constant  Value=3
  single_battery : Constant  Value=hvb.Bat2.cell.C_nom
  SB_BMS : Outport
  wires:
  Gain1/1 -> [OCV_Bat], Bus Creator/1  "V_Stackvoltage_V"
  n_bat_type_ID_i/1 -> Bus Creator/9  "n_bat_type_ID_i"
  b_Bat_available/1 -> Bus Creator/8  "b_Bat_available_b"
  Constant4/1 -> Bus Creator/7  "P_max_discharge_30s_W"
  Constant3/1 -> Bus Creator/6  "P_max_charge_30s_W"
  Constant2/1 -> Product2/2  "P_max_discharge_10s_W"
  Constant1/1 -> Product1/2  "P_max_charge_10s_W"
  Constant/1 -> Bus Creator/3  "t_max_currentPower_s"
  Bus Selector/5 -> [I_Bat_A], Terminator7/1, Product/1  "<Total_Current_A>"
  Bus Selector/4 -> MinMax2/1, MinMax1/1, Sum of Elements/1, Width/1  "<Voltage_Vector_V>"
  Bus Selector/3 -> " "/1, " "/1, MinMax/1, MinMax3/1  "<T_cell_degC>"
  Bus Selector/1 -> Gain1/1, Product/2  "<Total_Voltage_V>"
  Divide/1 -> Terminator6/1
  Width/1 -> Divide/2
  Sum of Elements/1 -> Divide/1
  MinMax3/1 -> Temp Regulation/1(T_max), Terminator4/1
  MinMax2/1 -> Terminator2/1
  MinMax1/1 -> Terminator3/1
  MinMax/1 -> Terminator5/1
  Gain/1 -> 1-D Lookup Table/1, 1-D Lookup Table1/1, Bus Creator/2  "SOC_perc"
  Bus Creator/1 -> SB_BMS/1
  PB_Bat/1 -> Bus Selector/1
  Product/1 -> Bus Creator/10  "P_currentPower_W"
  Unit Delay/1 -> Saturation Dynamic/2
  [OCV_Bat] -> Bus Creator/12  "Pack_OCV"
  Saturation Dynamic/1 -> Terminator1/1  "Ri_Bat_eq"
  Gain5/1 -> Divide1/2
  " "/1 -> Divide1/1
  [V_Stack_V] -> " "/2
  [OCV_Bat] -> " "/1
  [I_Bat_A] -> Gain5/1
  Divide1/1 -> Unit Delay/1
  [I_Bat_A] -> Bus Creator/13  "I_Bat_A"
  Gain4/1 -> Saturation Dynamic/3  "Pack_Ri_min"
  Ri/1 -> Gain4/1
  Gain3/1 -> Terminator/1  "Pack_OCV"
  Gain2/1 -> Saturation Dynamic/1  "Pack_Ri_max"
  " "/1 -> Ri/1, Bus Creator/14, 2-D Lookup Table1/1, Total_R/1  "T_Cell_avg"
  2-D Lookup Table1/1 -> Gain3/1  "Cell_OCV"
  Total_R/1 -> Gain2/1
  Bus Selector/2 -> Ri/2, 2-D Lookup Table1/2, Total_R/2, Gain/1  "<SOC_Vector_Percent>"
  " "/1 -> " "/2
  " "/1 -> " "/1
  n_bat_type_ID_i1/1 -> Bus Creator/11  "Ri_Bat_eq"
  Product1/1 -> Bus Creator/4  "P_max_charge_10s_W"
  Product2/1 -> Bus Creator/5  "P_max_discharge_10s_W"
  1-D Lookup Table1/1 -> Product1/1
  1-D Lookup Table/1 -> Product2/1
  Temp Regulation/2(Forced Air Cooling on) -> Bus Creator/16  "Forced Air Cooling on"
  Temp Regulation/3(Forced Cooled Coolant Cooling on) -> Bus Creator/17  "Forced Cooled Coolant Cooling on"
  Fast charging on/1 -> Temp Regulation/2(Fast charging on)
  Temp Regulation/4(Active Heating on) -> Bus Creator/18  "Active Heating on"
  Temp Regulation/1(Compressor Power Factor) -> Bus Creator/15  "Compressor  Power Factor"
  Temp Regulation/5(Velocity Air) -> Bus Creator/19  "Velocity Air"
  bat2_wh/1 -> Scope1/1, Bus Creator/20  "bat2_Wh"
  single_battery/1 -> Scope/1, Bus Creator/21  "single_battery"
  Num_cells/1 -> Bus Creator/22

== system HVModAL_Fahrzeugmodell/HV-Batteries (Hvb)/Bat_2/Temp_model ==
  note: 0: No cooling
      | 1: Active Aircooling
      | 2: Refrigerant Cooling
      | 3: Liquid Cooling
      | 4:Passive Aircooling
  Q_dotLoss : Inport
  T_environment : Inport  Port=2
  ForcedAir Cooling on : Inport  Port=3
  Forced Cooled Coolant Cooling on : Inport  Port=4
  Active Heating on : Inport  Port=5
  Compressor Power Factor : Inport  Port=6
  Velocity Airstream : Inport  Port=7
  ActiveAirCoolingCompressor : Subsystem
  AmbientAir : Subsystem
  Cell : Subsystem
  Cooling system : Constant  Value=mask_cooling_method
  CoolingChannel : Subsystem
  Delay : Delay  DelayLength=1  InitialCondition=0
  Delay1 : Delay  DelayLength=1  InitialCondition=0
  LiquidCoolingCompressor : Subsystem
  Pack2cell : Gain  Gain=1/mask_Num_Zellen_el_ser/mask_Num_Zellen_el_par
  Q_dot Cells2CoolingSys+AmbAir : MultiPortSwitch  DataPortOrder=Zero-based contiguous  Inputs=5
  Q_dot Cells2AmbAir+ Q_dotCells2Refri : Sum
  Q_dotCells2AmbAir+ Q_dotCells2CoolingSys : Sum
  Q_dotCoolantCompr+ Q_dotPTC : Sum
  Q_dot_All_Compressors : Sum
  T_cell  avg : Outport
  Q_dot_ AllCompressors +PTC : Outport  Port=2
  wires:
  Cell/1(T_cell avg) -> T_cell  avg/1, CoolingChannel/2(T_cell avg [K]), AmbientAir/2(T_cell avg)
  T_environment/1 -> CoolingChannel/1(T_environment), AmbientAir/5(T_environment), Cell/2(T_environment)
  LiquidCoolingCompressor/1(Q_dot LiquidCoolingSystem) -> Q_dotCoolantCompr+ Q_dotPTC/1, CoolingChannel/3(Q_dot LiquidCoolingSystem)
  AmbientAir/1(Q_dotHousingDissipation AmbientAir2Environment) -> Delay/1
  ForcedAir Cooling on/1 -> ActiveAirCoolingCompressor/1(ForcedAir Cooling on)
  ActiveAirCoolingCompressor/1(Velocity Air) -> AmbientAir/3(Velocity Air [m/s])
  LiquidCoolingCompressor/2(Q_dot PTC Heater) -> Q_dotCoolantCompr+ Q_dotPTC/2, CoolingChannel/4(Q_dot PTC Heater)
  Q_dot Cells2CoolingSys+AmbAir/1 -> Pack2cell/1  "Q_dot Cells2CoolingSys+AmbAir"
  Cooling system/1 -> Q_dot Cells2CoolingSys+AmbAir/1
  AmbientAir/2(Q_dotCells2AmbientAir) -> Q_dot Cells2CoolingSys+AmbAir/6, Q_dotCells2AmbAir+ Q_dotCells2CoolingSys/1, Q_dot Cells2AmbAir+ Q_dotCells2Refri/1, Q_dot Cells2CoolingSys+AmbAir/3, Q_dot Cells2CoolingSys+AmbAir/2
  CoolingChannel/1(Q_dot Cells2Refri) -> Q_dot Cells2AmbAir+ Q_dotCells2Refri/2
  CoolingChannel/2(Q_dot Cells2CoolingSystem) -> Q_dotCells2AmbAir+ Q_dotCells2CoolingSys/2
  Q_dotLoss/1 -> Cell/3(Q_dot Loss Cell)
  Pack2cell/1 -> Cell/1(Q_dot Cell2CoolingSystem+AmbientAir)  "Q_dot SingleCell2CoolingSys+AmbAir"
  Delay/1 -> AmbientAir/1(Q_dotHousingDissipation AmbientAir2Environment1)
  Q_dotCells2AmbAir+ Q_dotCells2CoolingSys/1 -> Q_dot Cells2CoolingSys+AmbAir/5
  Q_dot Cells2AmbAir+ Q_dotCells2Refri/1 -> Q_dot Cells2CoolingSys+AmbAir/4
  AmbientAir/3(T_AmbientAir) -> Delay1/1
  Delay1/1 -> AmbientAir/6(T_AmbientAir2)
  Forced Cooled Coolant Cooling on/1 -> ActiveAirCoolingCompressor/2(Forced Cooled Coolant Cooling on), LiquidCoolingCompressor/1(Forced Cooled Coolant Cooling on)
  Active Heating on/1 -> LiquidCoolingCompressor/2(Active Heating on)
  Compressor Power Factor/1 -> ActiveAirCoolingCompressor/3(Compressor Power Factor), LiquidCoolingCompressor/3(Compressor Power Factor)
  Velocity Airstream/1 -> ActiveAirCoolingCompressor/4(Velocity Airstream)
  Q_dotCoolantCompr+ Q_dotPTC/1 -> Q_dot_All_Compressors/2
  Q_dot_All_Compressors/1 -> Q_dot_ AllCompressors +PTC/1
  ActiveAirCoolingCompressor/2(Q_dotActiveAirCooling) -> Q_dot_All_Compressors/1, AmbientAir/4(Q_dotActiveAirCooling)

== system HVModAL_Fahrzeugmodell/HV-DcDc_Converters (Hdc)/HV-DcDc_Converter_Slave/Control Unit1 ==
  Emg_Pdc_demand : Inport
  Emg_U_dcDemand : Inport  Port=2
  at_Junction : Inport  Port=3
  Emg_U_bat : Inport  Port=4
  case : Inport  Port=5
  Add : Sum  Inputs=+-
  Divide : Product  Inputs=*/
  ImaxInput : Constant  Value=max(DCDCname.Pout)/min(DCDCname.Vin)
  Logical Operator : Logic  Operator=OR  Inputs=4  AllPortsSameDT=off  OutDataTypeStr=boolean
  Max Temperature : Constant  Value=max(DCDCname.Temperature)
  PtotMax : Constant  Value=max(DCDCname.Pout)
  Relational Operator{,1..3} (4 alike) : RelationalOperator  Operator=>  OutDataTypeStr=boolean
  Saturation1 : Saturate  UpperLimit=1  LowerLimit=0
  Saturation2 : Saturate  UpperLimit=max(DCDCname.Pout)  LowerLimit=-max(DCDCname.Pout)
  Saturation3 : Saturate  UpperLimit=max(DCDCname.Pout)  LowerLimit=-max(DCDCname.Pout)
  Sum : Sum  Inputs=+
  Switch : Switch  Criteria=u2 ~= 0
  UmaxInput : Constant  Value=max(DCDCname.Vin)
  UmaxOutput : Constant  Value=max(DCDCname.Vout)
  UmaxOutput1 : Constant  Value=5
  Pdc_avail : Outport
  Error : Outport  Port=2
  Pmax : Outport  Port=3
  wires:
  Relational Operator2/1 -> Sum/1
  Relational Operator1/1 -> Logical Operator/3
  Relational Operator/1 -> Logical Operator/2
  Relational Operator3/1 -> Logical Operator/1
  ImaxInput/1 -> Relational Operator3/2
  Divide/1 -> Relational Operator3/1
  Emg_U_bat/1 -> Relational Operator/1, Divide/2
  Emg_Pdc_demand/1 -> Saturation3/1, Saturation2/1, Divide/1
  Max Temperature/1 -> Relational Operator2/2
  at_Junction/1 -> Relational Operator2/1
  Logical Operator/1 -> Error/1
  Emg_U_dcDemand/1 -> Relational Operator1/1
  UmaxInput/1 -> Relational Operator/2
  UmaxOutput/1 -> Relational Operator1/2
  PtotMax/1 -> Pmax/1
  Sum/1 -> Saturation1/1
  Saturation1/1 -> Logical Operator/4
  Saturation2/1 -> Switch/1
  Switch/1 -> Pdc_avail/1
  case/1 -> Add/1
  UmaxOutput1/1 -> Add/2
  Add/1 -> Switch/2
  Saturation3/1 -> Switch/3

== system HVModAL_Fahrzeugmodell/Traction Inverters (Tri)/Tri1/Calc_Pmech ==
  In1 : Inport
  In2 : Inport  Port=2
  Product : Product
  f->omega : Gain  Gain=2*pi
  Pmech : Outport
  wires:
  f->omega/1 -> Product/1
  Product/1 -> Pmech/1
  In1/1 -> f->omega/1
  In2/1 -> Product/2

== system HVModAL_Fahrzeugmodell/Traction Inverters (Tri)/Tri1/Control Unit ==
  at_Ambient : Inport
  Elm_I_abc : Inport  Port=2
  Veh_frq_RotorActual : Inport  Port=3
  Tel_demand : Inport  Port=4
  Elm_at_endWindingsMagnet : Inport  Port=5
  Dcl_U : Inport  Port=6
  Tri_at_Junction : Inport  Port=7
  2-D Lookup Ud=f (n,T,Temp) : Lookup_n-D  NumberOfTableDimensions=3  BreakpointsForDimension1=ELMname.n  BreakpointsForDimension2=ELMname.tq  BreakpointsForDimension3=ELMname.temp  Table=elm.elm1.Ud  RndMeth=Simplest  InputSameDT=on
  2-D Lookup Uq=f (n,T,Temp) : Lookup_n-D  NumberOfTableDimensions=3  BreakpointsForDimension1=ELMname.n  BreakpointsForDimension2=ELMname.tq  BreakpointsForDimension3=ELMname.temp  Table=elm.elm1.Uq  InternalRulePriority=Speed  RndMeth=Simplest  InputSameDT=on
  Abs : Abs
  Demux : Demux  Outputs=2
  Pmax_Elm : Constant  Value=elm.elm1.pwr_mech_max
  Terminator : Terminator
  Terminator1 : Terminator
  Terminator2 : Terminator
  Thermal Control : Subsystem
  U0 : Constant  Value=0
  U_abc : Mux
  frq 2 rpm : Gain  Gain=60
  "n -> fel" : Gain  Gain=elm.elm1.polepair/60  SaturateOnIntegerOverflow=on
  Tri_U_abc : Outport
  Pmax_elm : Outport  Port=2
  Pmax : Outport  Port=3
  wires:
  Tel_demand/1 -> U_abc/3, 2-D Lookup Ud=f (n,T,Temp)/2, 2-D Lookup Uq=f (n,T,Temp)/2
  U_abc/1 -> Tri_U_abc/1
  2-D Lookup Uq=f (n,T,Temp)/1 -> U_abc/2
  frq 2 rpm/1 -> Abs/1
  "n -> fel"/1 -> U_abc/4
  2-D Lookup Ud=f (n,T,Temp)/1 -> U_abc/1
  Veh_frq_RotorActual/1 -> frq 2 rpm/1
  Elm_at_endWindingsMagnet/1 -> Demux/1
  Demux/1 -> 2-D Lookup Uq=f (n,T,Temp)/3, 2-D Lookup Ud=f (n,T,Temp)/3
  Dcl_U/1 -> Terminator1/1
  Elm_I_abc/1 -> Terminator2/1
  Pmax_Elm/1 -> Pmax_elm/1
  Tri_at_Junction/1 -> Thermal Control/1(Tri_at_Junction)
  at_Ambient/1 -> Thermal Control/2(at_Ambient)
  Thermal Control/1(Pmax) -> Pmax/1
  Abs/1 -> 2-D Lookup Ud=f (n,T,Temp)/1, 2-D Lookup Uq=f (n,T,Temp)/1, "n -> fel"/1
  Demux/2 -> Terminator/1

== system HVModAL_Fahrzeugmodell/Traction Inverters (Tri)/Tri1/Loss Calculation ==
  Dcl_U : Inport
  Elm_at_endWindingsMagnet : Inport  Port=2
  Plosses_elm : Inport  Port=3
  Tel_demand : Inport  Port=4
  Pmech : Inport  Port=5
  Veh_frq_RotorActual : Inport  Port=6
  f_sw : Inport  Port=7
  at_Junction : Inport  Port=8
  2-D Lookup I1=f (n,T,Temp) : Lookup_n-D  NumberOfTableDimensions=3  BreakpointsForDimension1=ELMname.n  BreakpointsForDimension2=ELMname.tq  BreakpointsForDimension3=ELMname.temp  Table=ELMname.I1  InternalRulePriority=Speed  RndMeth=Simplest  InputSameDT=on
  2-D Lookup Ud=f (n,T,Temp) : Lookup_n-D  NumberOfTableDimensions=3  BreakpointsForDimension1=ELMname.n  BreakpointsForDimension2=ELMname.tq  BreakpointsForDimension3=ELMname.temp  Table=ELMname.Ud  InternalRulePriority=Speed  RndMeth=Simplest  InputSameDT=on
  2-D Lookup Uq=f (n,T,Temp) : Lookup_n-D  NumberOfTableDimensions=3  BreakpointsForDimension1=ELMname.n  BreakpointsForDimension2=ELMname.tq  BreakpointsForDimension3=ELMname.temp  Table=ELMname.Uq  InternalRulePriority=Speed  RndMeth=Simplest  InputSameDT=on
  2-D Lookup cosphi=f(n,T,Temp) : Lookup_n-D  NumberOfTableDimensions=3  BreakpointsForDimension1=ELMname.n  BreakpointsForDimension2=ELMname.tq  BreakpointsForDimension3=ELMname.temp  Table=ELMname.cosphi  InternalRulePriority=Speed  RndMeth=Simplest  InputSameDT=on
  Abs2 : Abs
  Abs3 : Abs
  B6C : lib_tri_B6C/B6C
  Demux : Demux  Outputs=2
  Divide : Product  Inputs=*/
  Divide1 : Product  Inputs=*/
  Math Function : Math  Operator=square  OutDataTypeStr=double  SaturateOnIntegerOverflow=on
  Math Function1 : Math  Operator=square  SaturateOnIntegerOverflow=on
  "Peak Phase -> RMS Line" : Gain  Gain=sqrt(3)/sqrt(2)
  Saturation : Saturate  UpperLimit=1  LowerLimit=0.000001
  Saturation1 : Saturate  UpperLimit=1  LowerLimit=0.00000001
  Sqrt : Sqrt  SaturateOnIntegerOverflow=on
  Sum : Sum  Inputs=|++
  Sum of Elements : Sum  Inputs=+
  Sum1 : Sum  Inputs=++|
  Sum2 : Sum  Inputs=++|
  Sum3 : Sum  Inputs=++|
  Switch_motgen : Switch  Criteria=u2 > Threshold
  Terminator3 : Terminator
  "fm -> rpm" : Gain  Gain=60
  "n -> fel" : Gain  Gain=ELMname.polepair/60
  Tri_P_dcLink : Outport
  Tri_fac_eta : Outport  Port=2
  Tri_P_PE_Losses : Outport  Port=3
  Tri_P_Add_Losses : Outport  Port=4
  Tri_fac_eta1 : Outport  Port=5
  Tri_fac_eta2 : Outport  Port=6
  wires:
  Plosses_elm/1 -> Sum/2
  Veh_frq_RotorActual/1 -> "fm -> rpm"/1
  "fm -> rpm"/1 -> 2-D Lookup I1=f (n,T,Temp)/1, 2-D Lookup Ud=f (n,T,Temp)/1, 2-D Lookup Uq=f (n,T,Temp)/1, "n -> fel"/1, 2-D Lookup cosphi=f(n,T,Temp)/1
  Tel_demand/1 -> 2-D Lookup Ud=f (n,T,Temp)/2, 2-D Lookup cosphi=f(n,T,Temp)/2, 2-D Lookup Uq=f (n,T,Temp)/2, 2-D Lookup I1=f (n,T,Temp)/2
  2-D Lookup cosphi=f(n,T,Temp)/1 -> B6C/3
  "n -> fel"/1 -> B6C/4
  Elm_at_endWindingsMagnet/1 -> Demux/1
  Demux/1 -> 2-D Lookup Ud=f (n,T,Temp)/3, 2-D Lookup I1=f (n,T,Temp)/3, 2-D Lookup Uq=f (n,T,Temp)/3, 2-D Lookup cosphi=f(n,T,Temp)/3
  Dcl_U/1 -> B6C/5
  2-D Lookup Ud=f (n,T,Temp)/1 -> Math Function/1
  2-D Lookup Uq=f (n,T,Temp)/1 -> Math Function1/1
  Math Function1/1 -> Sum3/2
  Math Function/1 -> Sum3/1
  Sum3/1 -> Sqrt/1
  Pmech/1 -> Sum/1
  Divide/1 -> Saturation/1
  Saturation/1 -> Tri_fac_eta1/1, Switch_motgen/1
  Divide1/1 -> Saturation1/1
  Saturation1/1 -> Switch_motgen/3, Tri_fac_eta2/1
  Switch_motgen/1 -> Tri_fac_eta/1
  Sum1/1 -> Abs2/1, Tri_P_dcLink/1
  Abs3/1 -> Divide1/2, Divide/1
  Abs2/1 -> Divide1/1, Divide/2
  B6C/1 -> Tri_P_PE_Losses/1, Sum of Elements/1
  Sqrt/1 -> "Peak Phase -> RMS Line"/1
  at_Junction/1 -> B6C/6
  f_sw/1 -> B6C/7
  2-D Lookup I1=f (n,T,Temp)/1 -> B6C/1
  "Peak Phase -> RMS Line"/1 -> B6C/2
  Sum/1 -> Abs3/1, Sum1/2, Switch_motgen/2
  Sum of Elements/1 -> Sum2/2
  Sum2/1 -> Sum1/1
  B6C/2 -> Sum2/1, Tri_P_Add_Losses/1
  Demux/2 -> Terminator3/1

== system HVModAL_Fahrzeugmodell/Traction Inverters (Tri)/Tri1/Loss Calculation measured ==
  Dcl_U : Inport
  Elm_at_endWindingsMagnet : Inport  Port=2
  Plosses_elm : Inport  Port=3
  Tel_demand : Inport  Port=4
  Pmech : Inport  Port=5
  Veh_frq_RotorActual : Inport  Port=6
  f_sw : Inport  Port=7
  at_Junction : Inport  Port=8
  2-D Lookup I1=f (n,T,Temp) : Lookup_n-D  BreakpointsForDimension1=torquevec  BreakpointsForDimension2=speedvec  BreakpointsForDimension3=elm.elm1.temp  Table=lossestable  InternalRulePriority=Speed  RndMeth=Simplest  InputSameDT=on
  Abs2 : Abs
  Abs3 : Abs
  Demux : Demux  Outputs=2
  Divide : Product  Inputs=*/
  Divide1 : Product  Inputs=*/
  Saturation : Saturate  UpperLimit=1  LowerLimit=0.000001
  Saturation1 : Saturate  UpperLimit=1  LowerLimit=0
  Sum : Sum  Inputs=|++
  Sum1 : Sum  Inputs=++|
  Switch_motgen : Switch  Criteria=u2 > Threshold
  Terminator{1..5} (5 alike) : Terminator
  "fm -> rpm" : Gain  Gain=60
  Tri_P_dcLink : Outport
  Tri_P_Losses : Outport  Port=2
  Tri_fac_eta : Outport  Port=3
  wires:
  Plosses_elm/1 -> Sum/2
  Veh_frq_RotorActual/1 -> "fm -> rpm"/1
  "fm -> rpm"/1 -> 2-D Lookup I1=f (n,T,Temp)/2
  Tel_demand/1 -> 2-D Lookup I1=f (n,T,Temp)/1
  Elm_at_endWindingsMagnet/1 -> Demux/1
  Demux/1 -> Terminator3/1
  Sum/1 -> Abs3/1, Sum1/2, Switch_motgen/2
  Pmech/1 -> Sum/1
  Divide/1 -> Saturation/1
  Saturation/1 -> Switch_motgen/1
  Divide1/1 -> Saturation1/1
  Saturation1/1 -> Switch_motgen/3
  Switch_motgen/1 -> Tri_fac_eta/1
  Sum1/1 -> Abs2/1, Tri_P_dcLink/1
  Abs3/1 -> Divide1/2, Divide/1
  Abs2/1 -> Divide1/1, Divide/2
  2-D Lookup I1=f (n,T,Temp)/1 -> Sum1/1, Tri_P_Losses/1
  Demux/2 -> Terminator1/1
  Dcl_U/1 -> Terminator2/1
  at_Junction/1 -> Terminator4/1
  f_sw/1 -> Terminator5/1
